simulink library "RateBasedLib"  (Simulink 7.7)
settings: Solver=ode45  SolverMode=SingleTasking  StartTime=0.0  StopTime=10.0  RelTol=1e-3
undefined symbols (not defined in the file or in its folder): Faster, SF
libraries: RateBasedLib x1
settings Model: Creator=jpalma  LastModifiedBy=jpalma

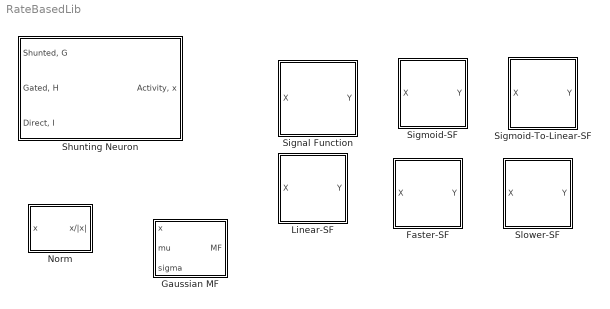
== system RateBasedLib ==
  Faster-SF : Subsystem
      mask Description: Author: Jesse Palma
      mask Help: Author: Jesse Palma
      mask Display: image(imread('../libs/icons/FasterSF.jpg'),'center');
  Gaussian MF : Subsystem  mask(gaussmf){sigma=1, mu=0}
      mask prompts: sigma "Variance sigma:"; mu "Mean c:"
      mask help:
      | Symmetric Gaussian membership function given by
      |
      |         f ( x ) = exp ^ ( ( - 0.5 ( x - c) ^ 2 ) / sigma ^ 2 )
      |
      | where c is the mean and sigma is the variance.
      mask init:
      | x=0:0.02:1;
      | params=[0.1 0.6];
      | y=gaussmf(x,params);
      mask Help: helpview(fullfile(docroot,'toolbox','fuzzy','fuzzy.map'), 'gaussmf');
      mask Display: plot(x,y);
  Linear-SF : Subsystem
      mask Description: Author: Jesse Palma
      mask Help: Author: Jesse Palma
      mask Display: image(imread('../libs/icons/LinearSF.jpg'),'center');
  Norm : Subsystem
      mask Description: blah blah
  Shunting Neuron : Subsystem  mask{A=0.1, B=1, tau=1}
      mask prompts: A "A, Decay Rate"; B "B, Shunting Max"; tau "tau, Time Constant"
      mask help:
      | This implements a neuron with activity (rate) x which decays at rate A.
      |
      | dx_i/dt = -Ax_i + G(B-x_i) + Hx_i + I
      |
      | Author: Jesse Palma
      mask Help:
      | This implements a neuron with activity (rate) x which decays at rate A.
      | 
      | dx_i/dt = -Ax_i + G(B-x_i) + Hx_i + I
      | 
      | Author: Jesse Palma
      mask Display: image(imread('../libs/icons/RateBased.jpg'),'center');
  Sigmoid-SF : Subsystem  mask{threshold=0.5, slope=8, asymptote=1, ground=0}
      mask help: Author: Jesse Palma
      mask Help: Author: Jesse Palma
      mask Display: image(imread('../libs/icons/SigmoidSF.jpg'),'center');
  Sigmoid-To-Linear-SF : Subsystem  mask{threshold=0.4, threshold2=0.55, slope=8, asymptote=0.73, ground=-0.025}
      mask prompts: threshold2 "Threshold of Switch"
      mask help: Author: Jesse Palma
      mask Help: Author: Jesse Palma
      mask Display: image(imread('../libs/icons/FasterLSF.jpg'),'center');
  Signal Function : Subsystem  BlockChoice=Faster-SF
      settings: TemplateBlock=self  MemberBlocks=Faster-SF,Linear-SF,Sigmoid-SF,Sigmoid-To-Linear-SF,Slower-SF
  Slower-SF : Subsystem
      mask Description: Author: Jesse Palma
      mask Help: Author: Jesse Palma
      mask Display: image(imread('../libs/icons/SlowerSF.jpg'),'center');

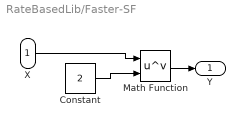
== system RateBasedLib/Faster-SF ==
  X : Inport
  Constant : Constant  Value=2
  Math Function : Math  Operator=pow  SaturateOnIntegerOverflow=on
  Y : Outport
  wires:
  Constant/1 -> Math Function/2
  Math Function/1 -> Y/1
  X/1 -> Math Function/1

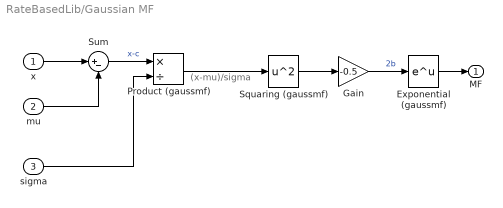
== system RateBasedLib/Gaussian MF ==
  note: (x-mu)/sigma
  x : Inport
  mu : Inport  Port=2
  sigma : Inport  Port=3
  Exponential (gaussmf) : Math  SaturateOnIntegerOverflow=on
  Gain : Gain  Gain=-0.5  SaturateOnIntegerOverflow=on  OutDataTypeStr=Inherit: Same as input  ParamDataTypeStr=Inherit: Same as input
  Product (gaussmf) : Product  Inputs=*/  SaturateOnIntegerOverflow=on  InputSameDT=on  OutDataTypeStr=Inherit: Same as first input
  Squaring (gaussmf) : Math  Operator=square  SaturateOnIntegerOverflow=on
  Sum : Sum  Inputs=|+-  SaturateOnIntegerOverflow=on  InputSameDT=on  OutDataTypeStr=Inherit: Same as first input
  MF : Outport
  wires:
  x/1 -> Sum/1
  mu/1 -> Sum/2
  Sum/1 -> Product (gaussmf)/1  "x-c"
  sigma/1 -> Product (gaussmf)/2
  Exponential (gaussmf)/1 -> MF/1
  Squaring (gaussmf)/1 -> Gain/1
  Gain/1 -> Exponential (gaussmf)/1  "2b"
  Product (gaussmf)/1 -> Squaring (gaussmf)/1

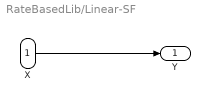
== system RateBasedLib/Linear-SF ==
  X : Inport
  Y : Outport
  wires:
  X/1 -> Y/1

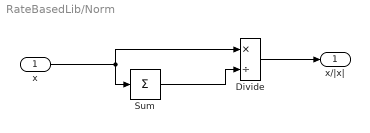
== system RateBasedLib/Norm ==
  x : Inport
  Divide : Product  Inputs=*/
  Sum : Sum  Inputs=+
  x/|x| : Outport
  wires:
  Divide/1 -> x/|x|/1
  x/1 -> Sum/1, Divide/1
  Sum/1 -> Divide/2

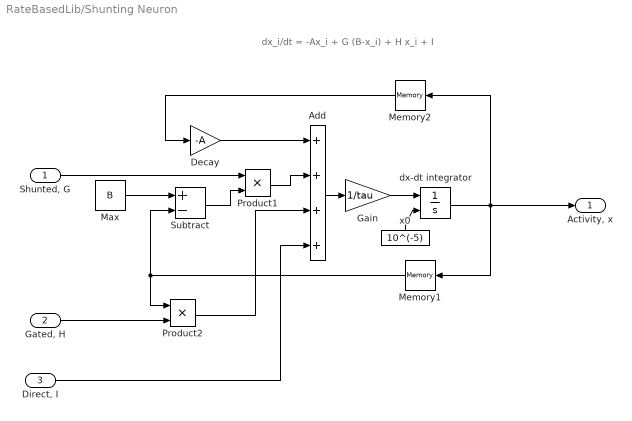
== system RateBasedLib/Shunting Neuron ==
  note: dx_i/dt = -Ax_i + G (B-x_i) + H x_i + I
  "Shunted, G" : Inport
  "Gated, H" : Inport  Port=2
  "Direct, I" : Inport  Port=3
  Add : Sum  Inputs=++++
  Decay : Gain  Gain=-A
  Gain : Gain  Gain=1/tau
  Max : Constant  Value=B
  Memory1 : Memory
  Memory2 : Memory
  Product1 : Product  RndMeth=Zero
  Product2 : Product  RndMeth=Zero
  Subtract : Sum  Inputs=+-
  dx-dt integrator : Integrator  InitialConditionSource=external
  x0 : Constant  Value=10^(-5)
  "Activity, x" : Outport
  wires:
  Memory2/1 -> Decay/1
  x0/1 -> dx-dt integrator/2
  Max/1 -> Subtract/1
  Subtract/1 -> Product1/2
  dx-dt integrator/1 -> "Activity, x"/1, Memory2/1, Memory1/1
  Add/1 -> Gain/1
  "Gated, H"/1 -> Product2/2
  Decay/1 -> Add/1
  Product1/1 -> Add/2
  Memory1/1 -> Subtract/2, Product2/1
  Product2/1 -> Add/3
  "Direct, I"/1 -> Add/4
  "Shunted, G"/1 -> Product1/1
  Gain/1 -> dx-dt integrator/1

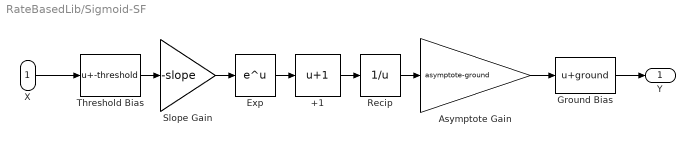
== system RateBasedLib/Sigmoid-SF ==
  X : Inport
  +1 : Bias  Bias=1
  Asymptote Gain : Gain  Gain=asymptote-ground
  Exp : Math  SaturateOnIntegerOverflow=on
  Ground Bias : Bias  Bias=ground
  Recip : Math  Operator=reciprocal  SaturateOnIntegerOverflow=on
  Slope Gain : Gain  Gain=-slope
  Threshold Bias : Bias  Bias=-threshold
  Y : Outport
  wires:
  Ground Bias/1 -> Y/1
  Asymptote Gain/1 -> Ground Bias/1
  X/1 -> Threshold Bias/1
  Recip/1 -> Asymptote Gain/1
  +1/1 -> Recip/1
  Exp/1 -> +1/1
  Slope Gain/1 -> Exp/1
  Threshold Bias/1 -> Slope Gain/1

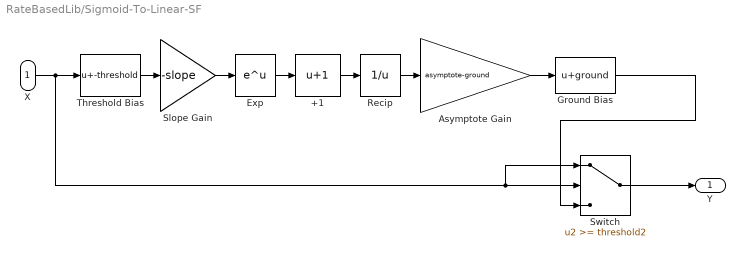
== system RateBasedLib/Sigmoid-To-Linear-SF ==
  X : Inport
  +1 : Bias  Bias=1
  Asymptote Gain : Gain  Gain=asymptote-ground
  Exp : Math  SaturateOnIntegerOverflow=on
  Ground Bias : Bias  Bias=ground
  Recip : Math  Operator=reciprocal  SaturateOnIntegerOverflow=on
  Slope Gain : Gain  Gain=-slope
  Switch : Switch  Threshold=threshold2
  Threshold Bias : Bias  Bias=-threshold
  Y : Outport
  wires:
  Threshold Bias/1 -> Slope Gain/1
  Slope Gain/1 -> Exp/1
  Exp/1 -> +1/1
  +1/1 -> Recip/1
  Recip/1 -> Asymptote Gain/1
  X/1 -> Threshold Bias/1, Switch/2, Switch/1
  Asymptote Gain/1 -> Ground Bias/1
  Switch/1 -> Y/1
  Ground Bias/1 -> Switch/3

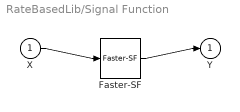
== system RateBasedLib/Signal Function ==
  X : Inport
  Faster-SF : RateBasedLib/Faster-SF  SystemSampleTime=-1
  Y : Outport
  wires:
  X/1 -> Faster-SF/1
  Faster-SF/1 -> Y/1

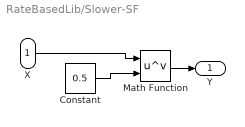
== system RateBasedLib/Slower-SF ==
  X : Inport
  Constant : Constant  Value=0.5
  Math Function : Math  Operator=pow  SaturateOnIntegerOverflow=on
  Y : Outport
  wires:
  X/1 -> Math Function/1
  Math Function/1 -> Y/1
  Constant/1 -> Math Function/2
